simulink model "Simscape_Actuated_Robot"  (R2025b)
settings: Solver=VariableStepAuto  StartTime=0.0  StopTime=20  RelTol=1e-3
InitFcn:
  | run("init.m");
values from neighbouring files (symbols this model uses):
  q_init = [pi/6,-pi/3, 0,pi/6,-pi/3,0]    [init.m]
undefined symbols (not defined in the file or in its folder): robot_params, X, Y, Z
libraries: sm_lib x48, nesl_utility x48
(part 2 of 2)

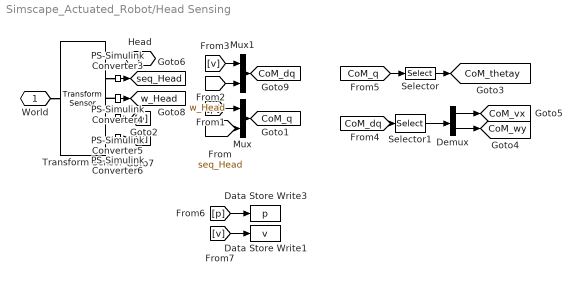
== system Simscape_Actuated_Robot/Head Sensing ==
  Data Store Write1 : DataStoreWrite  DataStoreName=v  DataStoreElements=v  EnableIndexing=on  NumberOfDimensions=2  IndexOptions=Index vector (dialog),Index vector (dialog)  Indices=[1 2 3],[2]  OutputSizes=1,1
  Data Store Write3 : DataStoreWrite  DataStoreName=p  DataStoreElements=p  EnableIndexing=on  NumberOfDimensions=2  IndexOptions=Index vector (dialog),Index vector (dialog)  Indices=[1 2 3],[1]  OutputSizes=1,1
  Demux : Demux  Outputs=2
  Mux : Mux  Inputs=2
  Mux1 : Mux  Inputs=2
  PS-Simulink Converter{3..6} (4 alike) : nesl_utility/PS-Simulink Converter  PhysicalDomain=network_engine_domain  SubClassName=ps_output  LeftPortType=input  RightPortType=output  PseudoPeriodic=off  Frequencies=[]  VectorFormat=inherit  Unit=inherit  AffineConversion=off
  Selector : Selector  InputPortWidth=6  IndexOptions=Index vector (dialog)  Indices=5  OutputSizes=1
  Selector1 : Selector  InputPortWidth=6  IndexOptions=Index vector (dialog)  Indices=[1 5]  OutputSizes=1
  Transform Sensor : sm_lib/Frames and Transforms/Transform Sensor  MeasurementFrame=World  RotationSequence=XYZ  SenseAngle=off  SenseAxis=off  SenseQ=off  SenseR=off  SenseRotationSequence=on  SenseOmegaX=off  SenseOmegaY=off  SenseOmegaZ=off  SenseOmega=on  SenseQDot=off  SenseRDot=off  SenseRotationSequenceDot=off  SenseAlphaX=off  SenseAlphaY=off  SenseAlphaZ=off  SenseAlpha=off  SenseQDDot=off  SenseRDDot=off  SenseX=off  SenseY=off  SenseZ=off  SenseXYZ=on  SenseRad=off  SenseAzim=off  SenseDist=off  SenseInc=off  SenseXDot=off  SenseYDot=off  SenseZDot=off  SenseXYZDot=on  SenseRadDot=off  SenseAzimDot=off  SenseDistDot=off  SenseIncDot=off  SenseXDDot=off  SenseYDDot=off  SenseZDDot=off  SenseXYZDDot=off  SenseRadDDot=off  SenseAzimDDot=off  SenseDistDDot=off  SenseIncDDot=off
  World : PMIOPort  Side=Right
  Head : PMIOPort  Port=2  Side=Left
  tag scope: CoM_dq=global, CoM_q=global, CoM_thetay=global, CoM_vx=global, CoM_wy=global, seq_Head=global, w_Head=global
  wires:
  Selector/1 -> [CoM_thetay]
  PS-Simulink Converter5/1 -> [p]
  PS-Simulink Converter3/1 -> [seq_Head]
  [p] -> Mux/1
  [seq_Head] -> Mux/2
  PS-Simulink Converter6/1 -> [v]
  PS-Simulink Converter4/1 -> [w_Head]
  Mux/1 -> [CoM_q]
  Mux1/1 -> [CoM_dq]
  [w_Head] -> Mux1/2
  [v] -> Mux1/1
  [CoM_dq] -> Selector1/1
  Selector1/1 -> Demux/1
  Demux/1 -> [CoM_vx]
  Demux/2 -> [CoM_wy]
  [CoM_q] -> Selector/1
  [p] -> Data Store Write3/1
  [v] -> Data Store Write1/1
  connections:
  PS-Simulink Converter6/LConn1 -- Transform Sensor/RConn5
  PS-Simulink Converter5/LConn1 -- Transform Sensor/RConn4
  PS-Simulink Converter4/LConn1 -- Transform Sensor/RConn3
  Transform Sensor/RConn2 -- PS-Simulink Converter3/LConn1
  Transform Sensor/RConn1 -- Head/RConn1
  World/RConn1 -- Transform Sensor/LConn1

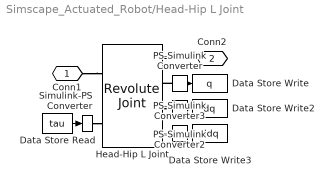
== system Simscape_Actuated_Robot/Head-Hip L Joint  ==
  Data Store Read : DataStoreRead  DataStoreName=tau  DataStoreElements=tau  EnableIndexing=on  IndexOptions=Index vector (dialog)  Indices=4  OutputSizes=1
  Data Store Write : DataStoreWrite  DataStoreName=q  DataStoreElements=q  EnableIndexing=on  IndexOptions=Index vector (dialog)  Indices=4  OutputSizes=1
  Data Store Write2 : DataStoreWrite  DataStoreName=dq  DataStoreElements=dq  EnableIndexing=on  IndexOptions=Index vector (dialog)  Indices=4  OutputSizes=1
  Data Store Write3 : DataStoreWrite  DataStoreName=ddq  DataStoreElements=ddq  EnableIndexing=on  IndexOptions=Index vector (dialog)  Indices=4  OutputSizes=1
  "Head-Hip L Joint " : sm_lib/Joints/Revolute Joint  JointMode=Normal  CompositeWrenchDir=FollowerOnBase  CompositeWrenchFrame=BaseFrame  SenseConstraintForce=off  SenseConstraintTorque=off  SenseTotalForce=off  SenseTotalTorque=off  PositionTargetSpecify=on  PositionTargetPriority=High  PositionTargetValue=q_init(4)  PositionTargetValueUnits=rad  VelocityTargetSpecify=off  VelocityTargetPriority=High  VelocityTargetValue=0  VelocityTargetValueUnits=rad/s  EquilibriumPosition=0  EquilibriumPositionUnits=rad  SpringStiffness=Motor_stiffness  SpringStiffnessUnits=N*m/deg  DampingCoefficient=Motor_damping  DampingCoefficientUnits=N*m/(deg/s)  LowerLimitSpecify=off  LowerLimitBound=-90  LowerLimitBoundUnits=deg  LowerLimitStiffness=1e4  LowerLimitStiffnessUnits=N*m/deg  LowerLimitDamping=10  LowerLimitDampingUnits=N*m/(deg/s)  LowerLimitTransitionRegionWidth=0.1  LowerLimitTransitionRegionWidthUnits=deg  UpperLimitSpecify=off  UpperLimitBound=90  UpperLimitBoundUnits=deg  UpperLimitStiffness=1e4  UpperLimitStiffnessUnits=N*m/deg  UpperLimitDamping=10  UpperLimitDampingUnits=N*m/(deg/s)  UpperLimitTransitionRegionWidth=0.1  UpperLimitTransitionRegionWidthUnits=deg  TorqueActuationMode=InputTorque  MotionActuationMode=ComputedMotion  SensePosition=on  SenseVelocity=on  SenseAcceleration=on  SenseTorqueForce=off  SenseLowerLimitTorqueForce=off  SenseUpperLimitTorqueForce=off
  PS-Simulink Converter : nesl_utility/PS-Simulink Converter  PhysicalDomain=network_engine_domain  SubClassName=ps_output  LeftPortType=input  RightPortType=output  PseudoPeriodic=off  Frequencies=[]  VectorFormat=1-D array  Unit=rad  AffineConversion=off
  PS-Simulink Converter2 : nesl_utility/PS-Simulink Converter  PhysicalDomain=network_engine_domain  SubClassName=ps_output  LeftPortType=input  RightPortType=output  PseudoPeriodic=off  Frequencies=[]  VectorFormat=1-D array  Unit=rad/s  AffineConversion=off
  PS-Simulink Converter3 : nesl_utility/PS-Simulink Converter  PhysicalDomain=network_engine_domain  SubClassName=ps_output  LeftPortType=input  RightPortType=output  PseudoPeriodic=off  Frequencies=[]  VectorFormat=inherit  Unit=inherit  AffineConversion=off
  Simulink-PS Converter : nesl_utility/Simulink-PS Converter  PhysicalDomain=network_engine_domain  SubClassName=ps_input  LeftPortType=input  RightPortType=output  PseudoPeriodic=off  Frequencies=[]  NoiseDistribution=none  NoiseParameters=[]  Unit=N*m  AffineConversion=off  FilteringAndDerivatives=provide  SimscapeFilterOrder=1  InputFilterTimeConstant=0.001  UdotUserProvided=0
  Conn1 : PMIOPort  Side=Left
  Conn2 : PMIOPort  Port=2  Side=Right
  wires:
  PS-Simulink Converter/1 -> Data Store Write/1
  PS-Simulink Converter2/1 -> Data Store Write2/1
  PS-Simulink Converter3/1 -> Data Store Write3/1
  Data Store Read/1 -> Simulink-PS Converter/1
  connections:
  Conn2/RConn1 -- "Head-Hip L Joint "/RConn1
  Conn1/RConn1 -- "Head-Hip L Joint "/LConn1
  PS-Simulink Converter/LConn1 -- "Head-Hip L Joint "/RConn2
  "Head-Hip L Joint "/RConn3 -- PS-Simulink Converter2/LConn1
  "Head-Hip L Joint "/RConn4 -- PS-Simulink Converter3/LConn1
  Simulink-PS Converter/RConn1 -- "Head-Hip L Joint "/LConn2

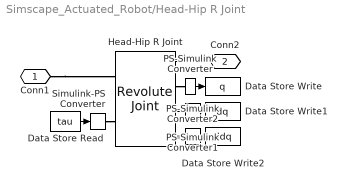
== system Simscape_Actuated_Robot/Head-Hip R Joint  ==
  Data Store Read : DataStoreRead  DataStoreName=tau  DataStoreElements=tau  EnableIndexing=on  IndexOptions=Index vector (dialog)  Indices=1  OutputSizes=1
  Data Store Write : DataStoreWrite  DataStoreName=q  DataStoreElements=q  EnableIndexing=on  IndexOptions=Index vector (dialog)  Indices=1  OutputSizes=1
  Data Store Write1 : DataStoreWrite  DataStoreName=dq  DataStoreElements=dq  EnableIndexing=on  IndexOptions=Index vector (dialog)  Indices=1  OutputSizes=1
  Data Store Write2 : DataStoreWrite  DataStoreName=ddq  DataStoreElements=ddq  EnableIndexing=on  IndexOptions=Index vector (dialog)  Indices=1  OutputSizes=1
  "Head-Hip R Joint " : sm_lib/Joints/Revolute Joint  JointMode=Normal  CompositeWrenchDir=FollowerOnBase  CompositeWrenchFrame=BaseFrame  SenseConstraintForce=off  SenseConstraintTorque=off  SenseTotalForce=off  SenseTotalTorque=off  PositionTargetSpecify=on  PositionTargetPriority=High  PositionTargetValue=q_init(1)  PositionTargetValueUnits=rad  VelocityTargetSpecify=off  VelocityTargetPriority=High  VelocityTargetValue=0  VelocityTargetValueUnits=deg/s  EquilibriumPosition=0  EquilibriumPositionUnits=rad  SpringStiffness=Motor_stiffness  SpringStiffnessUnits=N*m/deg  DampingCoefficient=Motor_damping  DampingCoefficientUnits=N*m/(deg/s)  LowerLimitSpecify=off  LowerLimitBound=-90  LowerLimitBoundUnits=deg  LowerLimitStiffness=1e4  LowerLimitStiffnessUnits=N*m/deg  LowerLimitDamping=10  LowerLimitDampingUnits=N*m/(deg/s)  LowerLimitTransitionRegionWidth=0.1  LowerLimitTransitionRegionWidthUnits=deg  UpperLimitSpecify=off  UpperLimitBound=90  UpperLimitBoundUnits=deg  UpperLimitStiffness=1e4  UpperLimitStiffnessUnits=N*m/deg  UpperLimitDamping=10  UpperLimitDampingUnits=N*m/(deg/s)  UpperLimitTransitionRegionWidth=0.1  UpperLimitTransitionRegionWidthUnits=deg  TorqueActuationMode=InputTorque  MotionActuationMode=ComputedMotion  SensePosition=on  SenseVelocity=on  SenseAcceleration=on  SenseTorqueForce=off  SenseLowerLimitTorqueForce=off  SenseUpperLimitTorqueForce=off
  PS-Simulink Converter : nesl_utility/PS-Simulink Converter  PhysicalDomain=network_engine_domain  SubClassName=ps_output  LeftPortType=input  RightPortType=output  PseudoPeriodic=off  Frequencies=[]  VectorFormat=1-D array  Unit=rad  AffineConversion=off
  PS-Simulink Converter1 : nesl_utility/PS-Simulink Converter  PhysicalDomain=network_engine_domain  SubClassName=ps_output  LeftPortType=input  RightPortType=output  PseudoPeriodic=off  Frequencies=[]  VectorFormat=1-D array  Unit=rad/s  AffineConversion=off
  PS-Simulink Converter2 : nesl_utility/PS-Simulink Converter  PhysicalDomain=network_engine_domain  SubClassName=ps_output  LeftPortType=input  RightPortType=output  PseudoPeriodic=off  Frequencies=[]  VectorFormat=1-D array  Unit=inherit  AffineConversion=off
  Simulink-PS Converter : nesl_utility/Simulink-PS Converter  PhysicalDomain=network_engine_domain  SubClassName=ps_input  LeftPortType=input  RightPortType=output  PseudoPeriodic=off  Frequencies=[]  NoiseDistribution=none  NoiseParameters=[]  Unit=N*m  AffineConversion=off  FilteringAndDerivatives=provide  SimscapeFilterOrder=1  InputFilterTimeConstant=0.001  UdotUserProvided=0
  Conn1 : PMIOPort  Side=Left
  Conn2 : PMIOPort  Port=2  Side=Right
  wires:
  PS-Simulink Converter/1 -> Data Store Write/1
  PS-Simulink Converter1/1 -> Data Store Write1/1
  PS-Simulink Converter2/1 -> Data Store Write2/1
  Data Store Read/1 -> Simulink-PS Converter/1
  connections:
  PS-Simulink Converter1/LConn1 -- "Head-Hip R Joint "/RConn3
  Conn2/RConn1 -- "Head-Hip R Joint "/RConn1
  "Head-Hip R Joint "/RConn2 -- PS-Simulink Converter/LConn1
  Conn1/RConn1 -- "Head-Hip R Joint "/LConn1
  PS-Simulink Converter2/LConn1 -- "Head-Hip R Joint "/RConn4
  Simulink-PS Converter/RConn1 -- "Head-Hip R Joint "/LConn2

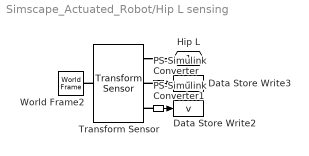
== system Simscape_Actuated_Robot/Hip L sensing ==
  Data Store Write2 : DataStoreWrite  DataStoreName=v  DataStoreElements=v  EnableIndexing=on  NumberOfDimensions=2  IndexOptions=Index vector (dialog),Index vector (dialog)  Indices=[1 2 3],[4]  OutputSizes=1,1
  Data Store Write3 : DataStoreWrite  DataStoreName=p  DataStoreElements=p  EnableIndexing=on  NumberOfDimensions=2  IndexOptions=Index vector (dialog),Index vector (dialog)  Indices=[1 2 3],[4]  OutputSizes=1,1
  PS-Simulink Converter : nesl_utility/PS-Simulink Converter  PhysicalDomain=network_engine_domain  SubClassName=ps_output  LeftPortType=input  RightPortType=output  PseudoPeriodic=off  Frequencies=[]  VectorFormat=inherit  Unit=inherit  AffineConversion=off
  PS-Simulink Converter1 : nesl_utility/PS-Simulink Converter  PhysicalDomain=network_engine_domain  SubClassName=ps_output  LeftPortType=input  RightPortType=output  PseudoPeriodic=off  Frequencies=[]  VectorFormat=inherit  Unit=inherit  AffineConversion=off
  Transform Sensor : sm_lib/Frames and Transforms/Transform Sensor  MeasurementFrame=World  RotationSequence=XYX  SenseAngle=off  SenseAxis=off  SenseQ=off  SenseR=off  SenseRotationSequence=off  SenseOmegaX=off  SenseOmegaY=off  SenseOmegaZ=off  SenseOmega=off  SenseQDot=off  SenseRDot=off  SenseRotationSequenceDot=off  SenseAlphaX=off  SenseAlphaY=off  SenseAlphaZ=off  SenseAlpha=off  SenseQDDot=off  SenseRDDot=off  SenseX=off  SenseY=off  SenseZ=off  SenseXYZ=on  SenseRad=off  SenseAzim=off  SenseDist=off  SenseInc=off  SenseXDot=off  SenseYDot=off  SenseZDot=off  SenseXYZDot=on  SenseRadDot=off  SenseAzimDot=off  SenseDistDot=off  SenseIncDot=off  SenseXDDot=off  SenseYDDot=off  SenseZDDot=off  SenseXYZDDot=off  SenseRadDDot=off  SenseAzimDDot=off  SenseDistDDot=off  SenseIncDDot=off
  World Frame2 : sm_lib/Frames and Transforms/World Frame
  Hip L : PMIOPort  Side=Right
  wires:
  PS-Simulink Converter/1 -> Data Store Write3/1
  PS-Simulink Converter1/1 -> Data Store Write2/1
  connections:
  PS-Simulink Converter/LConn1 -- Transform Sensor/RConn2
  Transform Sensor/RConn1 -- Hip L/RConn1
  Transform Sensor/LConn1 -- World Frame2/RConn1
  PS-Simulink Converter1/LConn1 -- Transform Sensor/RConn3

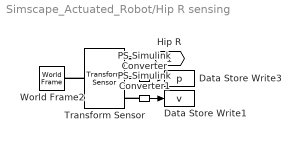
== system Simscape_Actuated_Robot/Hip R sensing ==
  Data Store Write1 : DataStoreWrite  DataStoreName=v  DataStoreElements=v  EnableIndexing=on  NumberOfDimensions=2  IndexOptions=Index vector (dialog),Index vector (dialog)  Indices=[1 2 3],[2]  OutputSizes=1,1
  Data Store Write3 : DataStoreWrite  DataStoreName=p  DataStoreElements=p  EnableIndexing=on  NumberOfDimensions=2  IndexOptions=Index vector (dialog),Index vector (dialog)  Indices=[1 2 3],[2]  OutputSizes=1,1
  PS-Simulink Converter : nesl_utility/PS-Simulink Converter  PhysicalDomain=network_engine_domain  SubClassName=ps_output  LeftPortType=input  RightPortType=output  PseudoPeriodic=off  Frequencies=[]  VectorFormat=inherit  Unit=inherit  AffineConversion=off
  PS-Simulink Converter1 : nesl_utility/PS-Simulink Converter  PhysicalDomain=network_engine_domain  SubClassName=ps_output  LeftPortType=input  RightPortType=output  PseudoPeriodic=off  Frequencies=[]  VectorFormat=inherit  Unit=inherit  AffineConversion=off
  Transform Sensor : sm_lib/Frames and Transforms/Transform Sensor  MeasurementFrame=World  RotationSequence=XYX  SenseAngle=off  SenseAxis=off  SenseQ=off  SenseR=off  SenseRotationSequence=off  SenseOmegaX=off  SenseOmegaY=off  SenseOmegaZ=off  SenseOmega=off  SenseQDot=off  SenseRDot=off  SenseRotationSequenceDot=off  SenseAlphaX=off  SenseAlphaY=off  SenseAlphaZ=off  SenseAlpha=off  SenseQDDot=off  SenseRDDot=off  SenseX=off  SenseY=off  SenseZ=off  SenseXYZ=on  SenseRad=off  SenseAzim=off  SenseDist=off  SenseInc=off  SenseXDot=off  SenseYDot=off  SenseZDot=off  SenseXYZDot=on  SenseRadDot=off  SenseAzimDot=off  SenseDistDot=off  SenseIncDot=off  SenseXDDot=off  SenseYDDot=off  SenseZDDot=off  SenseXYZDDot=off  SenseRadDDot=off  SenseAzimDDot=off  SenseDistDDot=off  SenseIncDDot=off
  World Frame2 : sm_lib/Frames and Transforms/World Frame
  Hip R : PMIOPort  Side=Right
  wires:
  PS-Simulink Converter/1 -> Data Store Write3/1
  PS-Simulink Converter1/1 -> Data Store Write1/1
  connections:
  Transform Sensor/LConn1 -- World Frame2/RConn1
  Transform Sensor/RConn1 -- Hip R/RConn1
  PS-Simulink Converter/LConn1 -- Transform Sensor/RConn2
  PS-Simulink Converter1/LConn1 -- Transform Sensor/RConn3

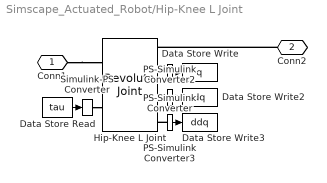
== system Simscape_Actuated_Robot/Hip-Knee L Joint ==
  Data Store Read : DataStoreRead  DataStoreName=tau  DataStoreElements=tau  EnableIndexing=on  IndexOptions=Index vector (dialog)  Indices=5  OutputSizes=1
  Data Store Write : DataStoreWrite  DataStoreName=q  DataStoreElements=q  EnableIndexing=on  IndexOptions=Index vector (dialog)  Indices=5  OutputSizes=1
  Data Store Write2 : DataStoreWrite  DataStoreName=dq  DataStoreElements=dq  EnableIndexing=on  IndexOptions=Index vector (dialog)  Indices=5  OutputSizes=1
  Data Store Write3 : DataStoreWrite  DataStoreName=ddq  DataStoreElements=ddq  EnableIndexing=on  IndexOptions=Index vector (dialog)  Indices=5  OutputSizes=1
  Hip-Knee L Joint : sm_lib/Joints/Revolute Joint  JointMode=Normal  CompositeWrenchDir=FollowerOnBase  CompositeWrenchFrame=BaseFrame  SenseConstraintForce=off  SenseConstraintTorque=off  SenseTotalForce=off  SenseTotalTorque=off  PositionTargetSpecify=on  PositionTargetPriority=High  PositionTargetValue=q_init(5)  PositionTargetValueUnits=rad  VelocityTargetSpecify=off  VelocityTargetPriority=High  VelocityTargetValue=0  VelocityTargetValueUnits=deg/s  EquilibriumPosition=0  EquilibriumPositionUnits=deg  SpringStiffness=Motor_stiffness  SpringStiffnessUnits=N*m/deg  DampingCoefficient=Motor_damping  DampingCoefficientUnits=N*m/(deg/s)  LowerLimitSpecify=off  LowerLimitBound=-90  LowerLimitBoundUnits=deg  LowerLimitStiffness=1e4  LowerLimitStiffnessUnits=N*m/deg  LowerLimitDamping=10  LowerLimitDampingUnits=N*m/(deg/s)  LowerLimitTransitionRegionWidth=0.1  LowerLimitTransitionRegionWidthUnits=deg  UpperLimitSpecify=off  UpperLimitBound=90  UpperLimitBoundUnits=deg  UpperLimitStiffness=1e4  UpperLimitStiffnessUnits=N*m/deg  UpperLimitDamping=10  UpperLimitDampingUnits=N*m/(deg/s)  UpperLimitTransitionRegionWidth=0.1  UpperLimitTransitionRegionWidthUnits=deg  TorqueActuationMode=InputTorque  MotionActuationMode=ComputedMotion  SensePosition=on  SenseVelocity=on  SenseAcceleration=on  SenseTorqueForce=off  SenseLowerLimitTorqueForce=off  SenseUpperLimitTorqueForce=off
  PS-Simulink Converter : nesl_utility/PS-Simulink Converter  PhysicalDomain=network_engine_domain  SubClassName=ps_output  LeftPortType=input  RightPortType=output  PseudoPeriodic=off  Frequencies=[]  VectorFormat=1-D array  Unit=rad  AffineConversion=off
  PS-Simulink Converter2 : nesl_utility/PS-Simulink Converter  PhysicalDomain=network_engine_domain  SubClassName=ps_output  LeftPortType=input  RightPortType=output  PseudoPeriodic=off  Frequencies=[]  VectorFormat=1-D array  Unit=rad/s  AffineConversion=off
  PS-Simulink Converter3 : nesl_utility/PS-Simulink Converter  PhysicalDomain=network_engine_domain  SubClassName=ps_output  LeftPortType=input  RightPortType=output  PseudoPeriodic=off  Frequencies=[]  VectorFormat=inherit  Unit=inherit  AffineConversion=off
  Simulink-PS Converter : nesl_utility/Simulink-PS Converter  PhysicalDomain=network_engine_domain  SubClassName=ps_input  LeftPortType=input  RightPortType=output  PseudoPeriodic=off  Frequencies=[]  NoiseDistribution=none  NoiseParameters=[]  Unit=N*m  AffineConversion=off  FilteringAndDerivatives=provide  SimscapeFilterOrder=1  InputFilterTimeConstant=0.001  UdotUserProvided=0
  Conn1 : PMIOPort  Side=Left
  Conn2 : PMIOPort  Port=2  Side=Right
  wires:
  PS-Simulink Converter/1 -> Data Store Write/1
  PS-Simulink Converter3/1 -> Data Store Write3/1
  PS-Simulink Converter2/1 -> Data Store Write2/1
  Data Store Read/1 -> Simulink-PS Converter/1
  connections:
  Conn2/RConn1 -- Hip-Knee L Joint/RConn1
  Conn1/RConn1 -- Hip-Knee L Joint/LConn1
  PS-Simulink Converter/LConn1 -- Hip-Knee L Joint/RConn2
  PS-Simulink Converter3/LConn1 -- Hip-Knee L Joint/RConn4
  PS-Simulink Converter2/LConn1 -- Hip-Knee L Joint/RConn3
  Simulink-PS Converter/RConn1 -- Hip-Knee L Joint/LConn2

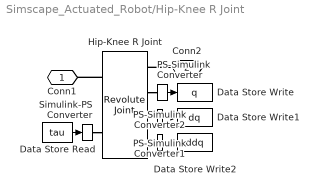
== system Simscape_Actuated_Robot/Hip-Knee R Joint ==
  Data Store Read : DataStoreRead  DataStoreName=tau  DataStoreElements=tau  EnableIndexing=on  IndexOptions=Index vector (dialog)  Indices=2  OutputSizes=1
  Data Store Write : DataStoreWrite  DataStoreName=q  DataStoreElements=q  EnableIndexing=on  IndexOptions=Index vector (dialog)  Indices=2  OutputSizes=1
  Data Store Write1 : DataStoreWrite  DataStoreName=dq  DataStoreElements=dq  EnableIndexing=on  IndexOptions=Index vector (dialog)  Indices=2  OutputSizes=1
  Data Store Write2 : DataStoreWrite  DataStoreName=ddq  DataStoreElements=ddq  EnableIndexing=on  IndexOptions=Index vector (dialog)  Indices=2  OutputSizes=1
  Hip-Knee R Joint : sm_lib/Joints/Revolute Joint  JointMode=Normal  CompositeWrenchDir=FollowerOnBase  CompositeWrenchFrame=BaseFrame  SenseConstraintForce=off  SenseConstraintTorque=off  SenseTotalForce=off  SenseTotalTorque=off  PositionTargetSpecify=on  PositionTargetPriority=High  PositionTargetValue=q_init(2)  PositionTargetValueUnits=rad  VelocityTargetSpecify=off  VelocityTargetPriority=High  VelocityTargetValue=0  VelocityTargetValueUnits=deg/s  EquilibriumPosition=0  EquilibriumPositionUnits=deg  SpringStiffness=Motor_stiffness  SpringStiffnessUnits=N*m/deg  DampingCoefficient=Motor_damping  DampingCoefficientUnits=N*m/(deg/s)  LowerLimitSpecify=off  LowerLimitBound=-90  LowerLimitBoundUnits=deg  LowerLimitStiffness=1e4  LowerLimitStiffnessUnits=N*m/deg  LowerLimitDamping=10  LowerLimitDampingUnits=N*m/(deg/s)  LowerLimitTransitionRegionWidth=0.1  LowerLimitTransitionRegionWidthUnits=deg  UpperLimitSpecify=off  UpperLimitBound=90  UpperLimitBoundUnits=deg  UpperLimitStiffness=1e4  UpperLimitStiffnessUnits=N*m/deg  UpperLimitDamping=10  UpperLimitDampingUnits=N*m/(deg/s)  UpperLimitTransitionRegionWidth=0.1  UpperLimitTransitionRegionWidthUnits=deg  TorqueActuationMode=InputTorque  MotionActuationMode=ComputedMotion  SensePosition=on  SenseVelocity=on  SenseAcceleration=on  SenseTorqueForce=off  SenseLowerLimitTorqueForce=off  SenseUpperLimitTorqueForce=off
  PS-Simulink Converter : nesl_utility/PS-Simulink Converter  PhysicalDomain=network_engine_domain  SubClassName=ps_output  LeftPortType=input  RightPortType=output  PseudoPeriodic=off  Frequencies=[]  VectorFormat=1-D array  Unit=rad  AffineConversion=off
  PS-Simulink Converter1 : nesl_utility/PS-Simulink Converter  PhysicalDomain=network_engine_domain  SubClassName=ps_output  LeftPortType=input  RightPortType=output  PseudoPeriodic=off  Frequencies=[]  VectorFormat=1-D array  Unit=rad/s  AffineConversion=off
  PS-Simulink Converter2 : nesl_utility/PS-Simulink Converter  PhysicalDomain=network_engine_domain  SubClassName=ps_output  LeftPortType=input  RightPortType=output  PseudoPeriodic=off  Frequencies=[]  VectorFormat=inherit  Unit=inherit  AffineConversion=off
  Simulink-PS Converter : nesl_utility/Simulink-PS Converter  PhysicalDomain=network_engine_domain  SubClassName=ps_input  LeftPortType=input  RightPortType=output  PseudoPeriodic=off  Frequencies=[]  NoiseDistribution=none  NoiseParameters=[]  Unit=N*m  AffineConversion=off  FilteringAndDerivatives=provide  SimscapeFilterOrder=1  InputFilterTimeConstant=0.001  UdotUserProvided=0
  Conn1 : PMIOPort  Side=Left
  Conn2 : PMIOPort  Port=2  Side=Right
  wires:
  PS-Simulink Converter/1 -> Data Store Write/1
  PS-Simulink Converter2/1 -> Data Store Write2/1
  PS-Simulink Converter1/1 -> Data Store Write1/1
  Data Store Read/1 -> Simulink-PS Converter/1
  connections:
  Conn2/RConn1 -- Hip-Knee R Joint/RConn1
  Hip-Knee R Joint/LConn1 -- Conn1/RConn1
  Hip-Knee R Joint/RConn2 -- PS-Simulink Converter/LConn1
  PS-Simulink Converter1/LConn1 -- Hip-Knee R Joint/RConn3
  PS-Simulink Converter2/LConn1 -- Hip-Knee R Joint/RConn4
  Simulink-PS Converter/RConn1 -- Hip-Knee R Joint/LConn2

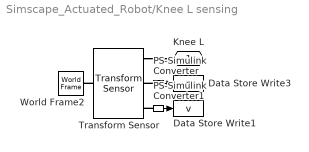
== system Simscape_Actuated_Robot/Knee L sensing ==
  Data Store Write1 : DataStoreWrite  DataStoreName=v  DataStoreElements=v  EnableIndexing=on  NumberOfDimensions=2  IndexOptions=Index vector (dialog),Index vector (dialog)  Indices=[1 2 3],[5]  OutputSizes=1,1
  Data Store Write3 : DataStoreWrite  DataStoreName=p  DataStoreElements=p  EnableIndexing=on  NumberOfDimensions=2  IndexOptions=Index vector (dialog),Index vector (dialog)  Indices=[1 2 3],[5]  OutputSizes=1,1
  PS-Simulink Converter : nesl_utility/PS-Simulink Converter  PhysicalDomain=network_engine_domain  SubClassName=ps_output  LeftPortType=input  RightPortType=output  PseudoPeriodic=off  Frequencies=[]  VectorFormat=inherit  Unit=inherit  AffineConversion=off
  PS-Simulink Converter1 : nesl_utility/PS-Simulink Converter  PhysicalDomain=network_engine_domain  SubClassName=ps_output  LeftPortType=input  RightPortType=output  PseudoPeriodic=off  Frequencies=[]  VectorFormat=inherit  Unit=inherit  AffineConversion=off
  Transform Sensor : sm_lib/Frames and Transforms/Transform Sensor  MeasurementFrame=World  RotationSequence=XYX  SenseAngle=off  SenseAxis=off  SenseQ=off  SenseR=off  SenseRotationSequence=off  SenseOmegaX=off  SenseOmegaY=off  SenseOmegaZ=off  SenseOmega=off  SenseQDot=off  SenseRDot=off  SenseRotationSequenceDot=off  SenseAlphaX=off  SenseAlphaY=off  SenseAlphaZ=off  SenseAlpha=off  SenseQDDot=off  SenseRDDot=off  SenseX=off  SenseY=off  SenseZ=off  SenseXYZ=on  SenseRad=off  SenseAzim=off  SenseDist=off  SenseInc=off  SenseXDot=off  SenseYDot=off  SenseZDot=off  SenseXYZDot=on  SenseRadDot=off  SenseAzimDot=off  SenseDistDot=off  SenseIncDot=off  SenseXDDot=off  SenseYDDot=off  SenseZDDot=off  SenseXYZDDot=off  SenseRadDDot=off  SenseAzimDDot=off  SenseDistDDot=off  SenseIncDDot=off
  World Frame2 : sm_lib/Frames and Transforms/World Frame
  Knee L : PMIOPort  Side=Right
  wires:
  PS-Simulink Converter/1 -> Data Store Write3/1
  PS-Simulink Converter1/1 -> Data Store Write1/1
  connections:
  Transform Sensor/LConn1 -- World Frame2/RConn1
  Transform Sensor/RConn1 -- Knee L/RConn1
  PS-Simulink Converter/LConn1 -- Transform Sensor/RConn2
  PS-Simulink Converter1/LConn1 -- Transform Sensor/RConn3

== system Simscape_Actuated_Robot/Knee R sensing ==
  Data Store Write1 : DataStoreWrite  DataStoreName=v  DataStoreElements=v  EnableIndexing=on  NumberOfDimensions=2  IndexOptions=Index vector (dialog),Index vector (dialog)  Indices=[1 2 3],[3]  OutputSizes=1,1
  Data Store Write3 : DataStoreWrite  DataStoreName=p  DataStoreElements=p  EnableIndexing=on  NumberOfDimensions=2  IndexOptions=Index vector (dialog),Index vector (dialog)  Indices=[1 2 3],[3]  OutputSizes=1,1
  PS-Simulink Converter : nesl_utility/PS-Simulink Converter  PhysicalDomain=network_engine_domain  SubClassName=ps_output  LeftPortType=input  RightPortType=output  PseudoPeriodic=off  Frequencies=[]  VectorFormat=inherit  Unit=inherit  AffineConversion=off
  PS-Simulink Converter1 : nesl_utility/PS-Simulink Converter  PhysicalDomain=network_engine_domain  SubClassName=ps_output  LeftPortType=input  RightPortType=output  PseudoPeriodic=off  Frequencies=[]  VectorFormat=inherit  Unit=inherit  AffineConversion=off
  Transform Sensor : sm_lib/Frames and Transforms/Transform Sensor  MeasurementFrame=World  RotationSequence=XYX  SenseAngle=off  SenseAxis=off  SenseQ=off  SenseR=off  SenseRotationSequence=off  SenseOmegaX=off  SenseOmegaY=off  SenseOmegaZ=off  SenseOmega=off  SenseQDot=off  SenseRDot=off  SenseRotationSequenceDot=off  SenseAlphaX=off  SenseAlphaY=off  SenseAlphaZ=off  SenseAlpha=off  SenseQDDot=off  SenseRDDot=off  SenseX=off  SenseY=off  SenseZ=off  SenseXYZ=on  SenseRad=off  SenseAzim=off  SenseDist=off  SenseInc=off  SenseXDot=off  SenseYDot=off  SenseZDot=off  SenseXYZDot=on  SenseRadDot=off  SenseAzimDot=off  SenseDistDot=off  SenseIncDot=off  SenseXDDot=off  SenseYDDot=off  SenseZDDot=off  SenseXYZDDot=off  SenseRadDDot=off  SenseAzimDDot=off  SenseDistDDot=off  SenseIncDDot=off
  World Frame2 : sm_lib/Frames and Transforms/World Frame
  Knee R : PMIOPort  Side=Right
  wires:
  PS-Simulink Converter/1 -> Data Store Write3/1
  PS-Simulink Converter1/1 -> Data Store Write1/1
  connections:
  PS-Simulink Converter/LConn1 -- Transform Sensor/RConn2
  Transform Sensor/RConn1 -- Knee R/RConn1
  Transform Sensor/LConn1 -- World Frame2/RConn1
  Transform Sensor/RConn3 -- PS-Simulink Converter1/LConn1

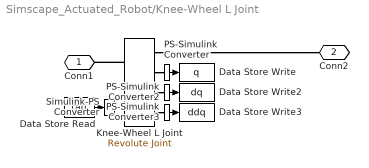
== system Simscape_Actuated_Robot/Knee-Wheel L Joint ==
  Data Store Read : DataStoreRead  DataStoreName=tau  DataStoreElements=tau  EnableIndexing=on  IndexOptions=Index vector (dialog)  Indices=6  OutputSizes=1
  Data Store Write : DataStoreWrite  DataStoreName=q  DataStoreElements=q  EnableIndexing=on  IndexOptions=Index vector (dialog)  Indices=6  OutputSizes=1
  Data Store Write2 : DataStoreWrite  DataStoreName=dq  DataStoreElements=dq  EnableIndexing=on  IndexOptions=Index vector (dialog)  Indices=6  OutputSizes=1
  Data Store Write3 : DataStoreWrite  DataStoreName=ddq  DataStoreElements=ddq  EnableIndexing=on  IndexOptions=Index vector (dialog)  Indices=6  OutputSizes=1
  Knee-Wheel L Joint : sm_lib/Joints/Revolute Joint  JointMode=Normal  CompositeWrenchDir=FollowerOnBase  CompositeWrenchFrame=BaseFrame  SenseConstraintForce=off  SenseConstraintTorque=off  SenseTotalForce=off  SenseTotalTorque=off  PositionTargetSpecify=on  PositionTargetPriority=High  PositionTargetValue=q_init(6)  PositionTargetValueUnits=rad  VelocityTargetSpecify=off  VelocityTargetPriority=High  VelocityTargetValue=0  VelocityTargetValueUnits=rad/s  EquilibriumPosition=0  EquilibriumPositionUnits=deg  SpringStiffness=Motor_stiffness  SpringStiffnessUnits=N*m/deg  DampingCoefficient=Motor_damping  DampingCoefficientUnits=N*m/(deg/s)  LowerLimitSpecify=off  LowerLimitBound=-90  LowerLimitBoundUnits=deg  LowerLimitStiffness=1e4  LowerLimitStiffnessUnits=N*m/deg  LowerLimitDamping=10  LowerLimitDampingUnits=N*m/(deg/s)  LowerLimitTransitionRegionWidth=0.1  LowerLimitTransitionRegionWidthUnits=deg  UpperLimitSpecify=off  UpperLimitBound=90  UpperLimitBoundUnits=deg  UpperLimitStiffness=1e4  UpperLimitStiffnessUnits=N*m/deg  UpperLimitDamping=10  UpperLimitDampingUnits=N*m/(deg/s)  UpperLimitTransitionRegionWidth=0.1  UpperLimitTransitionRegionWidthUnits=deg  TorqueActuationMode=InputTorque  MotionActuationMode=ComputedMotion  SensePosition=on  SenseVelocity=on  SenseAcceleration=on  SenseTorqueForce=off  SenseLowerLimitTorqueForce=off  SenseUpperLimitTorqueForce=off
  PS-Simulink Converter : nesl_utility/PS-Simulink Converter  PhysicalDomain=network_engine_domain  SubClassName=ps_output  LeftPortType=input  RightPortType=output  PseudoPeriodic=off  Frequencies=[]  VectorFormat=1-D array  Unit=rad  AffineConversion=off
  PS-Simulink Converter2 : nesl_utility/PS-Simulink Converter  PhysicalDomain=network_engine_domain  SubClassName=ps_output  LeftPortType=input  RightPortType=output  PseudoPeriodic=off  Frequencies=[]  VectorFormat=1-D array  Unit=rad/s  AffineConversion=off
  PS-Simulink Converter3 : nesl_utility/PS-Simulink Converter  PhysicalDomain=network_engine_domain  SubClassName=ps_output  LeftPortType=input  RightPortType=output  PseudoPeriodic=off  Frequencies=[]  VectorFormat=inherit  Unit=inherit  AffineConversion=off
  Simulink-PS Converter : nesl_utility/Simulink-PS Converter  PhysicalDomain=network_engine_domain  SubClassName=ps_input  LeftPortType=input  RightPortType=output  PseudoPeriodic=off  Frequencies=[]  NoiseDistribution=none  NoiseParameters=[]  Unit=N*m  AffineConversion=off  FilteringAndDerivatives=provide  SimscapeFilterOrder=1  InputFilterTimeConstant=0.001  UdotUserProvided=0
  Conn1 : PMIOPort  Side=Left
  Conn2 : PMIOPort  Port=2  Side=Right
  wires:
  PS-Simulink Converter3/1 -> Data Store Write3/1
  PS-Simulink Converter2/1 -> Data Store Write2/1
  PS-Simulink Converter/1 -> Data Store Write/1
  Data Store Read/1 -> Simulink-PS Converter/1
  connections:
  Knee-Wheel L Joint/RConn1 -- Conn2/RConn1
  Knee-Wheel L Joint/LConn1 -- Conn1/RConn1
  Knee-Wheel L Joint/RConn2 -- PS-Simulink Converter/LConn1
  Knee-Wheel L Joint/RConn3 -- PS-Simulink Converter2/LConn1
  Knee-Wheel L Joint/RConn4 -- PS-Simulink Converter3/LConn1
  Simulink-PS Converter/RConn1 -- Knee-Wheel L Joint/LConn2

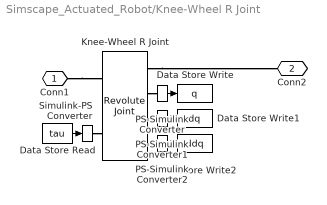
== system Simscape_Actuated_Robot/Knee-Wheel R Joint ==
  Data Store Read : DataStoreRead  DataStoreName=tau  DataStoreElements=tau  EnableIndexing=on  IndexOptions=Index vector (dialog)  Indices=3  OutputSizes=1
  Data Store Write : DataStoreWrite  DataStoreName=q  DataStoreElements=q  EnableIndexing=on  IndexOptions=Index vector (dialog)  Indices=3  OutputSizes=1
  Data Store Write1 : DataStoreWrite  DataStoreName=dq  DataStoreElements=dq  EnableIndexing=on  IndexOptions=Index vector (dialog)  Indices=3  OutputSizes=1
  Data Store Write2 : DataStoreWrite  DataStoreName=ddq  DataStoreElements=ddq  EnableIndexing=on  IndexOptions=Index vector (dialog)  Indices=3  OutputSizes=1
  Knee-Wheel R Joint : sm_lib/Joints/Revolute Joint  JointMode=Normal  CompositeWrenchDir=FollowerOnBase  CompositeWrenchFrame=BaseFrame  SenseConstraintForce=off  SenseConstraintTorque=off  SenseTotalForce=off  SenseTotalTorque=off  PositionTargetSpecify=on  PositionTargetPriority=High  PositionTargetValue=q_init(3)  PositionTargetValueUnits=deg  VelocityTargetSpecify=off  VelocityTargetPriority=High  VelocityTargetValue=q_init(3)  VelocityTargetValueUnits=rad/s  EquilibriumPosition=0  EquilibriumPositionUnits=deg  SpringStiffness=Motor_stiffness  SpringStiffnessUnits=N*m/deg  DampingCoefficient=Motor_damping  DampingCoefficientUnits=N*m/(deg/s)  LowerLimitSpecify=off  LowerLimitBound=-90  LowerLimitBoundUnits=deg  LowerLimitStiffness=1e4  LowerLimitStiffnessUnits=N*m/deg  LowerLimitDamping=10  LowerLimitDampingUnits=N*m/(deg/s)  LowerLimitTransitionRegionWidth=0.1  LowerLimitTransitionRegionWidthUnits=deg  UpperLimitSpecify=off  UpperLimitBound=90  UpperLimitBoundUnits=deg  UpperLimitStiffness=1e4  UpperLimitStiffnessUnits=N*m/deg  UpperLimitDamping=10  UpperLimitDampingUnits=N*m/(deg/s)  UpperLimitTransitionRegionWidth=0.1  UpperLimitTransitionRegionWidthUnits=deg  TorqueActuationMode=InputTorque  MotionActuationMode=ComputedMotion  SensePosition=on  SenseVelocity=on  SenseAcceleration=on  SenseTorqueForce=off  SenseLowerLimitTorqueForce=off  SenseUpperLimitTorqueForce=off
  PS-Simulink Converter : nesl_utility/PS-Simulink Converter  PhysicalDomain=network_engine_domain  SubClassName=ps_output  LeftPortType=input  RightPortType=output  PseudoPeriodic=off  Frequencies=[]  VectorFormat=1-D array  Unit=rad  AffineConversion=off
  PS-Simulink Converter1 : nesl_utility/PS-Simulink Converter  PhysicalDomain=network_engine_domain  SubClassName=ps_output  LeftPortType=input  RightPortType=output  PseudoPeriodic=off  Frequencies=[]  VectorFormat=1-D array  Unit=rad/s  AffineConversion=off
  PS-Simulink Converter2 : nesl_utility/PS-Simulink Converter  PhysicalDomain=network_engine_domain  SubClassName=ps_output  LeftPortType=input  RightPortType=output  PseudoPeriodic=off  Frequencies=[]  VectorFormat=inherit  Unit=inherit  AffineConversion=off
  Simulink-PS Converter : nesl_utility/Simulink-PS Converter  PhysicalDomain=network_engine_domain  SubClassName=ps_input  LeftPortType=input  RightPortType=output  PseudoPeriodic=off  Frequencies=[]  NoiseDistribution=none  NoiseParameters=[]  Unit=N*m  AffineConversion=off  FilteringAndDerivatives=provide  SimscapeFilterOrder=1  InputFilterTimeConstant=0.001  UdotUserProvided=0
  Conn1 : PMIOPort  Side=Left
  Conn2 : PMIOPort  Port=2  Side=Right
  wires:
  PS-Simulink Converter/1 -> Data Store Write/1
  PS-Simulink Converter1/1 -> Data Store Write1/1
  PS-Simulink Converter2/1 -> Data Store Write2/1
  Data Store Read/1 -> Simulink-PS Converter/1
  connections:
  Conn1/RConn1 -- Knee-Wheel R Joint/LConn1
  Knee-Wheel R Joint/RConn1 -- Conn2/RConn1
  Knee-Wheel R Joint/RConn2 -- PS-Simulink Converter/LConn1
  Knee-Wheel R Joint/RConn3 -- PS-Simulink Converter1/LConn1
  Knee-Wheel R Joint/RConn4 -- PS-Simulink Converter2/LConn1
  Simulink-PS Converter/RConn1 -- Knee-Wheel R Joint/LConn2

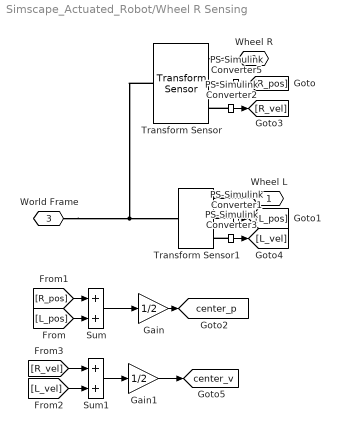
== system Simscape_Actuated_Robot/Wheel R Sensing ==
  Gain : Gain  Gain=1/2
  Gain1 : Gain  Gain=1/2
  PS-Simulink Converter{1..3,5} (4 alike) : nesl_utility/PS-Simulink Converter  PhysicalDomain=network_engine_domain  SubClassName=ps_output  LeftPortType=input  RightPortType=output  PseudoPeriodic=off  Frequencies=[]  VectorFormat=inherit  Unit=inherit  AffineConversion=off
  Sum : Sum
  Sum1 : Sum
  Transform Sensor : sm_lib/Frames and Transforms/Transform Sensor  MeasurementFrame=World  RotationSequence=XYZ  SenseAngle=off  SenseAxis=off  SenseQ=off  SenseR=off  SenseRotationSequence=off  SenseOmegaX=off  SenseOmegaY=off  SenseOmegaZ=off  SenseOmega=off  SenseQDot=off  SenseRDot=off  SenseRotationSequenceDot=off  SenseAlphaX=off  SenseAlphaY=off  SenseAlphaZ=off  SenseAlpha=off  SenseQDDot=off  SenseRDDot=off  SenseX=off  SenseY=off  SenseZ=off  SenseXYZ=on  SenseRad=off  SenseAzim=off  SenseDist=off  SenseInc=off  SenseXDot=off  SenseYDot=off  SenseZDot=off  SenseXYZDot=on  SenseRadDot=off  SenseAzimDot=off  SenseDistDot=off  SenseIncDot=off  SenseXDDot=off  SenseYDDot=off  SenseZDDot=off  SenseXYZDDot=off  SenseRadDDot=off  SenseAzimDDot=off  SenseDistDDot=off  SenseIncDDot=off
  Transform Sensor1 : sm_lib/Frames and Transforms/Transform Sensor  MeasurementFrame=World  RotationSequence=XYZ  SenseAngle=off  SenseAxis=off  SenseQ=off  SenseR=off  SenseRotationSequence=off  SenseOmegaX=off  SenseOmegaY=off  SenseOmegaZ=off  SenseOmega=off  SenseQDot=off  SenseRDot=off  SenseRotationSequenceDot=off  SenseAlphaX=off  SenseAlphaY=off  SenseAlphaZ=off  SenseAlpha=off  SenseQDDot=off  SenseRDDot=off  SenseX=off  SenseY=off  SenseZ=off  SenseXYZ=on  SenseRad=off  SenseAzim=off  SenseDist=off  SenseInc=off  SenseXDot=off  SenseYDot=off  SenseZDot=off  SenseXYZDot=on  SenseRadDot=off  SenseAzimDot=off  SenseDistDot=off  SenseIncDot=off  SenseXDDot=off  SenseYDDot=off  SenseZDDot=off  SenseXYZDDot=off  SenseRadDDot=off  SenseAzimDDot=off  SenseDistDDot=off  SenseIncDDot=off
  Wheel L : PMIOPort  Side=Left
  Wheel R : PMIOPort  Port=2  Side=Right
  "World Frame " : PMIOPort  Port=3  Side=Right
  tag scope: center_p=global, center_v=global
  wires:
  PS-Simulink Converter5/1 -> [R_pos]
  PS-Simulink Converter1/1 -> [L_pos]
  [R_pos] -> Sum/1
  [L_pos] -> Sum/2
  Sum/1 -> Gain/1
  Gain/1 -> [center_p]
  PS-Simulink Converter2/1 -> [R_vel]
  PS-Simulink Converter3/1 -> [L_vel]
  Sum1/1 -> Gain1/1
  [R_vel] -> Sum1/1
  [L_vel] -> Sum1/2
  Gain1/1 -> [center_v]
  connections:
  Transform Sensor/RConn1 -- Wheel R/RConn1
  "World Frame "/RConn1 -- Transform Sensor1/LConn1 -- Transform Sensor/LConn1
  PS-Simulink Converter5/LConn1 -- Transform Sensor/RConn2
  Wheel L/RConn1 -- Transform Sensor1/RConn1
  PS-Simulink Converter1/LConn1 -- Transform Sensor1/RConn2
  PS-Simulink Converter2/LConn1 -- Transform Sensor/RConn3
  PS-Simulink Converter3/LConn1 -- Transform Sensor1/RConn3

== matlab function Simscape_Actuated_Robot/MATLAB Function1 ==
  data: q input; tau output; dq input; v_ref input; dIv output; dW output; dg output; Iv input; W input; K parameter
function [tau, dIv, dW, dg] = SMC_control(q,      dq,      v_ref, Iv, W, K)


[tau, dIv, dW, dg] = wbr_ctrl(q,  dq, v_ref, Iv, W, K);

== matlab function Simscape_Actuated_Robot/MATLAB Function2 ==
  data: q input; tau output; dq input; v_ref input; dIv output; dW output; dg output; Iv input; W input; K parameter
function [tau, dIv, dW, dg] = SMC_control(q,      dq,      v_ref, Iv, W, K)


[tau, dIv, dW, dg] = wbr_ctrl(q,  dq, v_ref, Iv, W, K);

== matlab function Simscape_Actuated_Robot/MATLAB Function3 ==
  data: t input; s_des output; s_dot_des output
function [s_des, s_dot_des] = Smooth_Trajectory(t)
    % PRE-ALLOCAZIONE PER IL CODER
    s_des = 0.0;
    s_dot_des = 0.0;
    
    % PARAMETRI DELLA TRAIETTORIA
    t_start = .5;       % Il robot inizia a muoversi a 2 secondi
    t_end = 4.5;         % Arriva a destinazione a 5 secondi (3 secondi di viaggio)
    s_final = 1.0;       % Destinazione orizzontale (1 metro)
    
    % LOGICA DEL MOVIMENTO
    if t <= t_start
        % Prima di partire, resta fermo
        s_des = 0.0;
        s_dot_des = 0.0;
        
    elseif t >= t_end
        % Arrivato a destinazione, fermati
        s_des = s_final;
        s_dot_des = 0.0;
        
    else
        % FASE DI MOTO: Polinomio Cubico (Minimum Jerk Trajectory)
        % Normalizziamo il tempo tra 0 e 1 per la durata del viaggio
        tau = (t - t_start) / (t_end - t_start);
        
        % Posizione (Profilo a "S" morbida)
        s_des = s_final * (3*tau^2 - 2*tau^3);
        
        % Velocità (Derivata della posizione, forma a campana)
        s_dot_des = s_final * (6*tau - 6*tau^2) / (t_end - t_start);
    end
end

== matlab function Simscape_Actuated_Robot/MATLAB Function4 ==
  data: alpha output; CoM_p input; wx output; center_p input; CoM_v input; center_v input
function [alpha, wx] = fcn(CoM_p, center_p, CoM_v, center_v)
    % 1. Vettore posizione relativa (r) e velocità relativa (r_dot)
    r = CoM_p - center_p;
    r_dot = CoM_v - center_v;
    
    % 2. Estrazione delle componenti vettoriali per leggibilità (X=1, Y=2, Z=3)
    rx = r(1); 
    ry = r(2); 
    rz = r(3);
    
    rx_dot = r_dot(1); 
    ry_dot = r_dot(2); 
    rz_dot = r_dot(3);
    
    % 3. Calcolo del modulo (norma) del vettore r e la sua potenza al cubo
    norm_r = sqrt(rx^2 + ry^2 + rz^2);
    
    % 4. Calcolo del termine (rx*rx_dot + ry*ry_dot + rz*rz_dot) 
    % che corrisponde al prodotto scalare (dot product)
    dot_r = rx*rx_dot + ry*ry_dot + rz*rz_dot;
    
    % 5. Derivata dell'argomento della funzione: d/dt (rx / ||r||)
    d_arg = (rx_dot / norm_r) - (rx * dot_r) / norm_r.^3;
    
    % 6. Calcolo finale applicando la derivata dell'arcoseno per ottenere wx (ovvero alpha_dot)
    wx = (1 / sqrt(1 - (rx / norm_r)^2)) * d_arg;
    alpha = asin(rx./norm_r);

end
